simulink model "Salmuera2"  (R2021b)
settings: Solver=VariableStepAuto  StartTime=0.0  StopTime=5  RelTol=1e-3
settings Model: Creator=juandiegocastropadilla  LastModifiedBy=juandiegocastropadilla

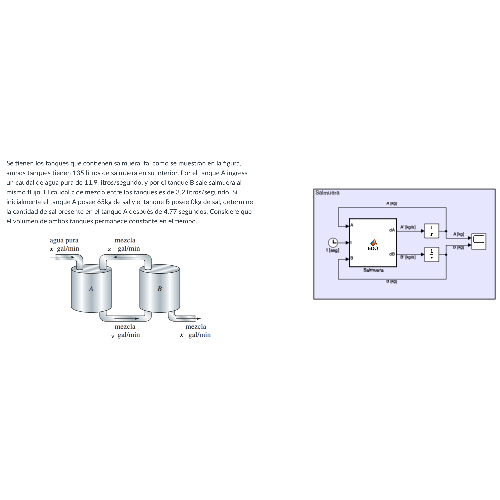
[thumbnail: Simulink's stored preview of the top-level diagram]
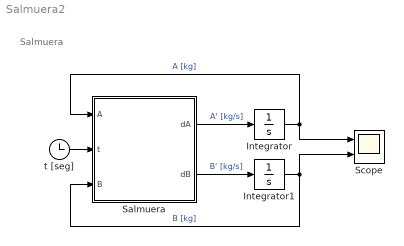
== system Salmuera2 ==
  note: Salmuera
  " Salmuera" : MATLAB Function  TreatAsAtomicUnit=on
  Integrator : Integrator  InitialCondition=65
  Integrator1 : Integrator
  Scope : Scope  NumInputPorts=2
  t [seg] : Clock
  wires:
  Integrator/1 -> Scope/1, " Salmuera"/1(A)  "A [kg]"
  Integrator1/1 -> " Salmuera"/3(B), Scope/2  "B [kg]"
  " Salmuera"/1(dA) -> Integrator/1  "A' [kg/s]"
  " Salmuera"/2(dB) -> Integrator1/1  "B' [kg/s]"
  t [seg]/1 -> " Salmuera"/2(t)

== matlab function Salmuera2/ Salmuera ==
  data: A input; t input; dA output; B input; dB output
function [dA, dB] = EDO(A, t, B)

x = 11.9; % L/s
y = 15.1; % L/s
z = 3.2;  % L/s 

VA0 = 135; % L
VB0 = 135; % L

VA = VA0 + t*(x+z-y); % L
VB = VB0 + t*(y-z-x); % L

cin = 0; % Kg/L

dA = x*(cin) + z*(B/VB) - y*(A/VA);
dB = y*(A/VA) - z*(B/VB) - x*(B/VB);
